simulink model "simulation_PI_controller"  (R2023a)
settings: Solver=VariableStepAuto  StartTime=0.0  StopTime=50  MaxStep=1e-3
settings Model: Creator=mazen  LastModifiedBy=mazen

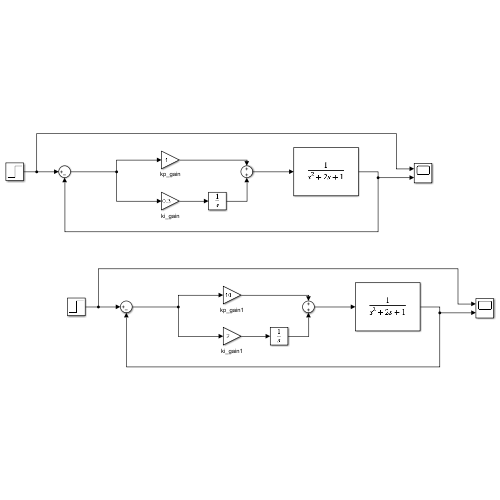
[thumbnail: Simulink's stored preview of the top-level diagram]
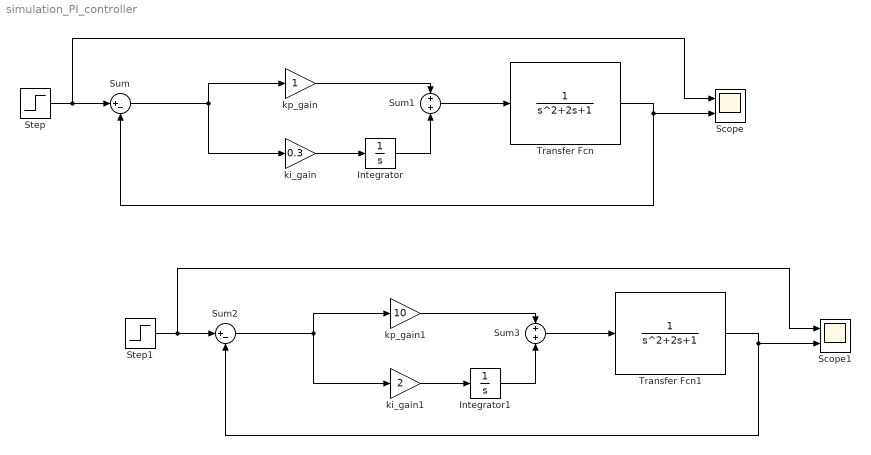
== system simulation_PI_controller ==
  Integrator : Integrator
  Integrator1 : Integrator
  Scope : Scope  NumInputPorts=2
  Scope1 : Scope  NumInputPorts=2
  Step : Step  SampleTime=0
  Step1 : Step  SampleTime=0
  Sum : Sum  Inputs=|+-
  Sum1 : Sum
  Sum2 : Sum  Inputs=|+-
  Sum3 : Sum
  Transfer Fcn : TransferFcn
  Transfer Fcn1 : TransferFcn
  ki_gain : Gain  Gain=0.3
  ki_gain1 : Gain  Gain=2
  kp_gain : Gain
  kp_gain1 : Gain  Gain=10
  wires:
  ki_gain/1 -> Integrator/1
  Sum/1 -> ki_gain/1, kp_gain/1
  kp_gain/1 -> Sum1/1
  Sum1/1 -> Transfer Fcn/1
  Integrator/1 -> Sum1/2
  Transfer Fcn/1 -> Sum/2, Scope/2
  Step/1 -> Scope/1, Sum/1
  Step1/1 -> Sum2/1, Scope1/1
  Transfer Fcn1/1 -> Scope1/2, Sum2/2
  Integrator1/1 -> Sum3/2
  Sum3/1 -> Transfer Fcn1/1
  kp_gain1/1 -> Sum3/1
  Sum2/1 -> kp_gain1/1, ki_gain1/1
  ki_gain1/1 -> Integrator1/1
